simulink model "gravity_comp_joint_space"  (R2023a)
settings: Solver=VariableStepAuto  StartTime=0.0  StopTime=5  RelTol=1e-3
undefined symbols (not defined in the file): dqi, g_d, gravity_on, KD, KP, noise, qd, qi, robot
settings Model: Creator=franc  LastModifiedBy=franc

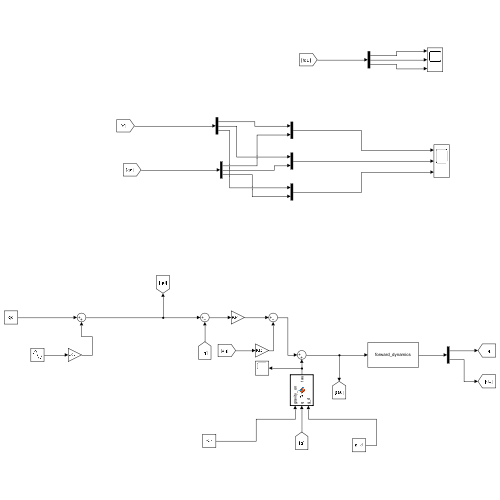
[thumbnail: Simulink's stored preview of the top-level diagram]
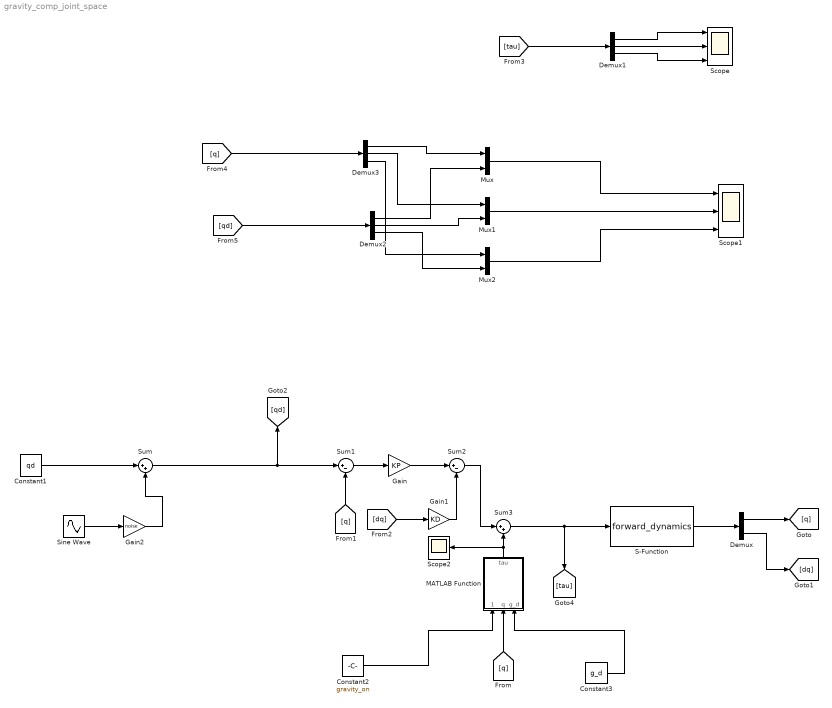
== system gravity_comp_joint_space ==
  Constant1 : Constant  Value=qd
  Constant2 : Constant  Value=gravity_on
  Constant3 : Constant  Value=g_d
  Demux : Demux  Outputs=2
  Demux1 : Demux  Outputs=3
  Demux2 : Demux  Outputs=3
  Demux3 : Demux  Outputs=3
  Gain : Gain  Gain=KP
  Gain1 : Gain  Gain=KD
  Gain2 : Gain  Gain=noise
  MATLAB Function : MATLAB Function  TreatAsAtomicUnit=on
  Mux : Mux  Inputs=2
  Mux1 : Mux  Inputs=2
  Mux2 : Mux  Inputs=2
  S-Function : S-Function  FunctionName=forward_dynamics  Parameters=robot,qi,dqi  SFunctionDeploymentMode=off  EnableBusSupport=off
  Scope : Scope  NumInputPorts=3
  Scope1 : Scope  NumInputPorts=3
  Scope2 : Scope
  Sine Wave : Sin  Amplitude=0.02  SampleTime=0
  Sum : Sum  Inputs=|++
  Sum1 : Sum  Inputs=|+-
  Sum2 : Sum  Inputs=|+-
  Sum3 : Sum  Inputs=|++
  wires:
  Sum1/1 -> Gain/1
  Gain/1 -> Sum2/1
  Sum3/1 -> S-Function/1, [tau]
  Gain1/1 -> Sum2/2
  Sum2/1 -> Sum3/1
  Demux/1 -> [q]
  S-Function/1 -> Demux/1
  Demux/2 -> [dq]
  [q] -> MATLAB Function/2(q)
  [q] -> Sum1/2
  [dq] -> Gain1/1
  MATLAB Function/1(tau) -> Scope2/1, Sum3/2
  [tau] -> Demux1/1
  Demux1/2 -> Scope/2
  Demux1/1 -> Scope/1
  Demux1/3 -> Scope/3
  [qd] -> Demux2/1
  Mux2/1 -> Scope1/3
  [q] -> Demux3/1
  Demux3/1 -> Mux/1
  Demux2/1 -> Mux/2
  Demux3/2 -> Mux1/1
  Demux3/3 -> Mux2/1
  Demux2/2 -> Mux1/2
  Demux2/3 -> Mux2/2
  Mux1/1 -> Scope1/2
  Mux/1 -> Scope1/1
  Constant2/1 -> MATLAB Function/1(gravity_on)
  Constant3/1 -> MATLAB Function/3(g_d)
  Sum/1 -> Sum1/1, [qd]
  Gain2/1 -> Sum/2
  Sine Wave/1 -> Gain2/1
  Constant1/1 -> Sum/1

== matlab function gravity_comp_joint_space/MATLAB Function ==
  data: gravity_on input; q input; tau output; g_d input
function tau = G(gravity_on, q,g_d)

    tau = zeros(3,1);

    if gravity_on == 1

        tau = get_G_as_9(q(1),q(2),q(3));
    end

    if gravity_on == 0

        tau = [0,0,0]';

    end
    if gravity_on == 2
        tau = g_d;

    end

end
